simulink model "sbw_data_flow_12_1"  (Simulink 5.0)
settings: Solver=ode45  StartTime=0.0  StopTime=10.0  RelTol=1e-3
settings Model: LastModifiedBy=sandeep

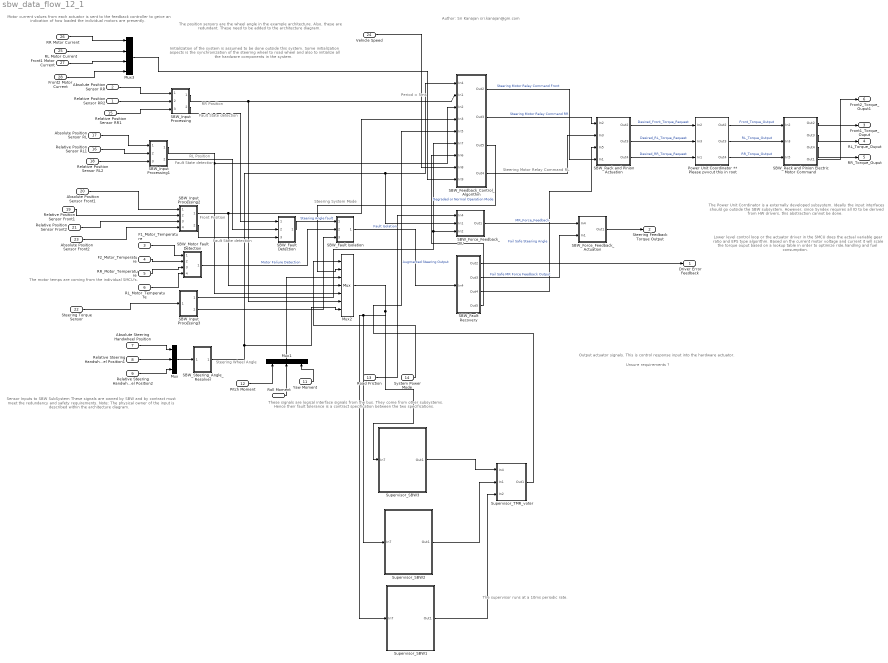
== system sbw_data_flow_12_1 ==
  note: The position sensors are the wheel angle in the example
      | architecture. Also, these are redundant. These need to be added to the architecture
      | diagram.
  note: Sensor Inputs to SBW SubSystem
      | These signals are owned by SBW and by
      | contract must meet the redundancy and safety requirements.
      | Note: The physical
      | owner of the input is described within
      | the architecture diagram.
  note: The motor temps
      | are coming from the
      | individual SMCU's.
  note: These signals are logical interface signals from the bus.
      | They come from other subsystems. Hence their fault tolerance
      | is a contract specification between the two specifications.
  note: Output actuator signals. This is control response
      | input into the hardware actuator.
  note: Steering Wheel Angle
  note: RR Position
  note: RL Position
  note: Front Position
  note: Fault State detection
  note: Fault State detection
  note: Fault State detection
  note: Steering System Mode
  note: Period = 5ms
  note: Steering Motor Relay Command RL
  note: Initialization of the system is assumed to be done outside this system.
      | Some initialization aspects is the synchronization of the steering wheel to
      | road wheel and also to initialize all the hardware components in the system.
  note: The Power Unit Corrdinator is a externally developed
      | subsystem. Ideally the input interfaces should go outside the SBW subsystem.
      | However, since Syndex requires all IO to be derived from HW drivers, this abstraction
      | cannot be done.
  note: Unsure requirements ?
  note: Lower level control loop or the actuator driver in the SMCU
      | does the actual variable gear ratio and EPS type algorithm. Based
      | on the current motor voltage and current it will scale the torque ouput based
      | on a lookup table in order to optimize ride,handling and fuel consumption.
  note: The supervisor runs at
      | a 10ms periodic rate.
  note: Motor current values from each
      | actuator is sent to the feedback controller
      | to geive an indication of how loaded the individual
      | motors are presently.
  note: Author: Sri Kanajan
      | sri.kanajan@gm.com
  Relative Position Sensor RR2 : Inport
  Absolute Position Sensor RR : Inport  Port=2
  F1_Motor_Temperature : Inport  Port=3
  F2_Motor_Temperature : Inport  Port=4
  RR_Motor_Temperature : Inport  Port=5
  RL_Motor_Temperature : Inport  Port=6
  Absolute Steering Handwheel Position : Inport  Port=7
  Relative Steering Handwheel Position1 : Inport  Port=8
  Relative Steering Handwheel Position2 : Inport  Port=9
  Roll Moment : Inport  Port=10
  Yaw Moment : Inport  Port=11
  Pitch Moment : Inport  Port=12
  Road Friction : Inport  Port=13
  System Power Mode : Inport  Port=14
  Relative Position Sensor RR1 : Inport  Port=15
  Relative Position Sensor RL1 : Inport  Port=16
  Absolute Position Sensor RL : Inport  Port=17
  Relative Position Sensor RL2 : Inport  Port=18
  Relative Position Sensor Front1 : Inport  Port=19
  Absolute Position Sensor Front1 : Inport  Port=20
  Relative Position Sensor Front2 : Inport  Port=21
  Steering Torque Sensor : Inport  Port=22
  Absolute Position Sensor Front2 : Inport  Port=23
  Vehicle Speed : Inport  Port=24
  RL Motor Current : Inport  Port=25
  RR Motor Current : Inport  Port=26
  Front1 Motor Current : Inport  Port=27
  Front2 Motor Current : Inport  Port=28
  Mux : Mux  Inputs=3
  Mux1 : Mux  Orientation=up  Inputs=3
  Mux2 : Mux  Inputs=7
  Mux3 : Mux
  Power Unit Coordinator ** Please pvvcut this in root : Subsystem
  SBW_Fault Detection : Subsystem
  SBW_Fault Isolation : Subsystem
  SBW_Fault Recovery : Subsystem
  SBW_Feedback_Control_Algorithm : Subsystem
  SBW_Force_Feedback_Actuation : Subsystem
  SBW_Force_Feedback_DIU : Subsystem
  SBW_Input Processing : Subsystem
  SBW_Input Processing1 : Subsystem
  SBW_Input Processing2 : Subsystem
  SBW_Input Processing3 : Subsystem
  SBW_Motor Fault Detection : Subsystem
  SBW_Rack and Pinion Actuation : Subsystem
  SBW_Rack and Pinion Electric Motor Command : Subsystem
  SBW_Steering_Angle_Resolver : Subsystem
  Supervisor_SBW1 : Subsystem
  Supervisor_SBW2 : Subsystem
  Supervisor_SBW3 : Subsystem
  Supervisor_TMR_voter : Subsystem
  Driver Error Feedback : Outport
  Steering Feedback Torque Output : Outport  Port=2
  Front1_Torque_Ouput : Outport  Port=3
  RL_Torque_Ouput : Outport  Port=4
  RR_Torque_Ouput : Outport  Port=5
  Front2_Torque_Ouput1 : Outport  Port=6
  wires:
  Absolute Steering Handwheel Position/1 -> Mux/1
  Relative Steering Handwheel Position1/1 -> Mux/2
  Relative Steering Handwheel Position2/1 -> Mux/3
  Absolute Position Sensor RR/1 -> SBW_Input Processing/1(In4)
  Relative Position Sensor RR2/1 -> SBW_Input Processing/2(In5)
  F1_Motor_Temperature/1 -> SBW_Motor Fault Detection/1(In4)
  F2_Motor_Temperature/1 -> SBW_Motor Fault Detection/2(In5)
  RR_Motor_Temperature/1 -> SBW_Motor Fault Detection/3(In1)
  RL_Motor_Temperature/1 -> SBW_Motor Fault Detection/4(In2)
  Mux/1 -> SBW_Steering_Angle_Resolver/1(In4)
  Relative Position Sensor RR1/1 -> SBW_Input Processing/3(In1)
  Absolute Position Sensor RL/1 -> SBW_Input Processing1/1(In4)
  Relative Position Sensor RL1/1 -> SBW_Input Processing1/2(In5)
  Relative Position Sensor RL2/1 -> SBW_Input Processing1/3(In1)
  Absolute Position Sensor Front1/1 -> SBW_Input Processing2/1(In4)
  Relative Position Sensor Front1/1 -> SBW_Input Processing2/2(In5)
  Relative Position Sensor Front2/1 -> SBW_Input Processing2/3(In1)
  SBW_Steering_Angle_Resolver/1(Out1) -> SBW_Feedback_Control_Algorithm/1(In4), SBW_Force_Feedback_DIU/2(In1), Mux2/7
  SBW_Input Processing/1(Out1) -> SBW_Feedback_Control_Algorithm/2(In1), Mux2/6
  SBW_Input Processing1/1(Out1) -> Mux2/5, SBW_Feedback_Control_Algorithm/3(In2)
  SBW_Input Processing2/1(Out1) -> SBW_Feedback_Control_Algorithm/4(In3), Mux2/4
  SBW_Force_Feedback_DIU/1(Out1) -> SBW_Force_Feedback_Actuation/1(In4)  "MR_Force_Feedback"
  SBW_Input Processing2/2(Out2) -> SBW_Fault Detection/3(In1)
  SBW_Input Processing/2(Out2) -> SBW_Fault Detection/1(In4)
  SBW_Input Processing1/2(Out2) -> SBW_Fault Detection/2(In5)
  Road Friction/1 -> SBW_Force_Feedback_DIU/1(In4)
  System Power Mode/1 -> Mux2/1
  SBW_Feedback_Control_Algorithm/2(Out3) -> SBW_Rack and Pinion Actuation/1(In2)  "Steering Motor Relay Command RR"
  SBW_Fault Detection/1(Out1) -> SBW_Fault Isolation/1(In4)  "Steering Angle fault"
  SBW_Motor Fault Detection/1(Out1) -> SBW_Fault Isolation/2(In5)  "Motor Faliure Detection"
  SBW_Fault Isolation/1(Out1) -> SBW_Fault Recovery/1(In4)  "Fault Isolation"
  SBW_Fault Recovery/1(Out2) -> Driver Error Feedback/1
  SBW_Feedback_Control_Algorithm/3(Out5) -> Mux2/2
  SBW_Fault Recovery/2(Out3) -> SBW_Force_Feedback_Actuation/2(In1)  "Fail Safe MR Force Feedback Output"
  SBW_Fault Recovery/3(Out4) -> SBW_Rack and Pinion Actuation/3(In5)  "Fail Safe Steering Angle"
  SBW_Force_Feedback_Actuation/1(Out1) -> Steering Feedback Torque Output/1
  SBW_Feedback_Control_Algorithm/4(Out4) -> SBW_Rack and Pinion Actuation/2(In3)
  SBW_Feedback_Control_Algorithm/1(Out2) -> SBW_Rack and Pinion Actuation/4(In1)  "Steering Motor Relay Command Front"
  SBW_Rack and Pinion Actuation/3(Out4) -> Power Unit Coordinator ** Please pvvcut this in root/3(In1)  "Desired_RR_Torque_Request"
  SBW_Rack and Pinion Actuation/2(Out3) -> Power Unit Coordinator ** Please pvvcut this in root/2(In3)  "Desired_RL_Torque_Request"
  SBW_Rack and Pinion Actuation/1(Out2) -> Power Unit Coordinator ** Please pvvcut this in root/1(In2)  "Desired_Front_Torque_Request"
  Power Unit Coordinator ** Please pvvcut this in root/2(Out3) -> SBW_Rack and Pinion Electric Motor Command/2(In3)  "RL_Torque_Output"
  Power Unit Coordinator ** Please pvvcut this in root/3(Out4) -> SBW_Rack and Pinion Electric Motor Command/3(In5)  "RR_Torque_Output"
  SBW_Rack and Pinion Electric Motor Command/1(Out2) -> Front1_Torque_Ouput/1
  Power Unit Coordinator ** Please pvvcut this in root/1(Out2) -> SBW_Rack and Pinion Electric Motor Command/1(In2)  "Front_Torque_Output"
  SBW_Rack and Pinion Electric Motor Command/2(Out3) -> RL_Torque_Ouput/1
  SBW_Rack and Pinion Electric Motor Command/3(Out4) -> RR_Torque_Ouput/1
  Absolute Position Sensor Front2/1 -> SBW_Input Processing2/4(In2)
  Pitch Moment/1 -> Mux1/1
  Roll Moment/1 -> Mux1/2
  Yaw Moment/1 -> Mux1/3
  Mux1/1 -> Mux2/3
  SBW_Rack and Pinion Electric Motor Command/4(Out1) -> Front2_Torque_Ouput1/1
  Mux2/1 -> Supervisor_SBW3/1(In7), Supervisor_SBW2/1(In7), Supervisor_SBW1/1(In7)
  Supervisor_SBW3/1(Out1) -> Supervisor_TMR_voter/1(In4)
  Supervisor_SBW2/1(Out1) -> Supervisor_TMR_voter/2(In1)
  Supervisor_SBW1/1(Out1) -> Supervisor_TMR_voter/3(In2)
  Supervisor_TMR_voter/1(Out1) -> SBW_Feedback_Control_Algorithm/5(In5)  "Augmented Steering Output"
  SBW_Fault Recovery/4(Out5) -> SBW_Feedback_Control_Algorithm/7(In6)  "Degraded or Normal Operation Mode"
  SBW_Input Processing3/1(Out1) -> SBW_Feedback_Control_Algorithm/6(In7), SBW_Force_Feedback_DIU/3(In2)
  SBW_Input Processing3/2(Out2) -> SBW_Fault Isolation/3(In1)
  Steering Torque Sensor/1 -> SBW_Input Processing3/1(In1)
  Vehicle Speed/1 -> SBW_Feedback_Control_Algorithm/8(In8)
  RR Motor Current/1 -> Mux3/1
  RL Motor Current/1 -> Mux3/2
  Front1 Motor Current/1 -> Mux3/3
  Front2 Motor Current/1 -> Mux3/4
  Mux3/1 -> SBW_Feedback_Control_Algorithm/9(In9)

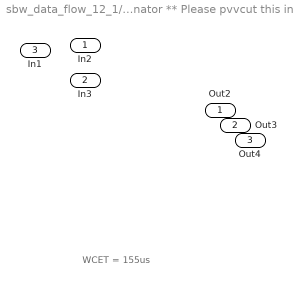
== system sbw_data_flow_12_1/Power Unit Coordinator ** Please pvvcut this in root ==
  note: WCET = 155us
  In2 : Inport
  In3 : Inport  Port=2
  In1 : Inport  Port=3
  Out2 : Outport
  Out3 : Outport  Port=2
  Out4 : Outport  Port=3

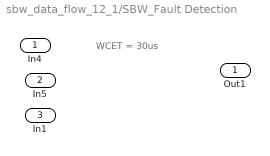
== system sbw_data_flow_12_1/SBW_Fault Detection ==
  note: WCET = 30us
  In4 : Inport
  In5 : Inport  Port=2
  In1 : Inport  Port=3
  Out1 : Outport

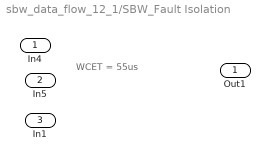
== system sbw_data_flow_12_1/SBW_Fault Isolation ==
  note: WCET = 55us
  In4 : Inport
  In5 : Inport  Port=2
  In1 : Inport  Port=3
  Out1 : Outport

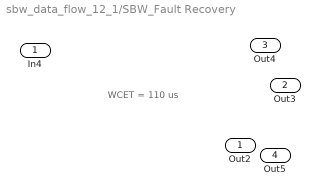
== system sbw_data_flow_12_1/SBW_Fault Recovery ==
  note: WCET = 110 us
  In4 : Inport
  Out2 : Outport
  Out3 : Outport  Port=2
  Out4 : Outport  Port=3
  Out5 : Outport  Port=4

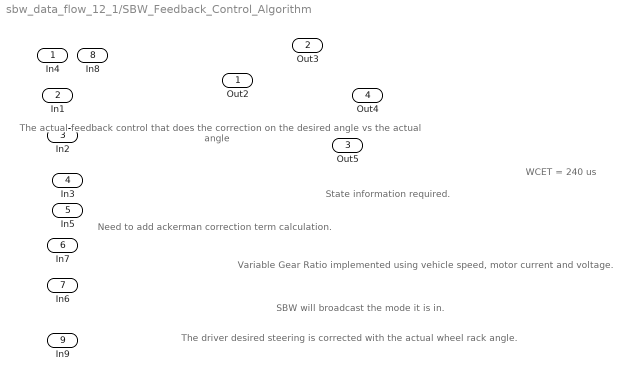
== system sbw_data_flow_12_1/SBW_Feedback_Control_Algorithm ==
  note: The actual feedback control
      | that does the correction on the
      | desired angle vs the actual angle
  note: Need to add ackerman correction
      | term calculation.
  note: State information required.
  note: WCET = 240 us
  note: SBW will broadcast the mode it is in.
  note: The driver desired steering is corrected
      | with the actual wheel rack angle.
  note: Variable Gear Ratio implemented using vehicle speed, motor current and voltage.
  In4 : Inport
  In1 : Inport  Port=2
  In2 : Inport  Port=3
  In3 : Inport  Port=4
  In5 : Inport  Port=5
  In7 : Inport  Port=6
  In6 : Inport  Port=7
  In8 : Inport  Port=8
  In9 : Inport  Port=9
  Out2 : Outport
  Out3 : Outport  Port=2
  Out5 : Outport  Port=3
  Out4 : Outport  Port=4

== system sbw_data_flow_12_1/SBW_Force_Feedback_Actuation ==
  note: WCET = 55us
  In4 : Inport
  In1 : Inport  Port=2
  Out1 : Outport

== system sbw_data_flow_12_1/SBW_Force_Feedback_DIU ==
  note: WCET = 190us
  In4 : Inport
  In1 : Inport  Port=2
  In2 : Inport  Port=3
  Out1 : Outport

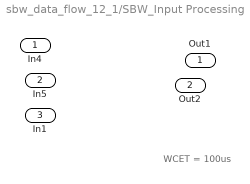
== system sbw_data_flow_12_1/SBW_Input Processing ==
  note: WCET = 100us
  In4 : Inport
  In5 : Inport  Port=2
  In1 : Inport  Port=3
  Out1 : Outport
  Out2 : Outport  Port=2

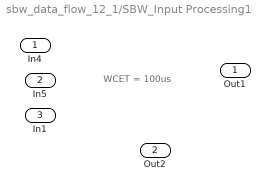
== system sbw_data_flow_12_1/SBW_Input Processing1 ==
  note: WCET = 100us
  In4 : Inport
  In5 : Inport  Port=2
  In1 : Inport  Port=3
  Out1 : Outport
  Out2 : Outport  Port=2

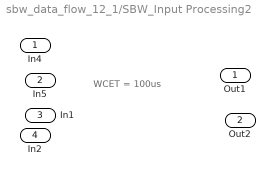
== system sbw_data_flow_12_1/SBW_Input Processing2 ==
  note: WCET = 100us
  In4 : Inport
  In5 : Inport  Port=2
  In1 : Inport  Port=3
  In2 : Inport  Port=4
  Out1 : Outport
  Out2 : Outport  Port=2

== system sbw_data_flow_12_1/SBW_Input Processing3 ==
  note: WCET = 100us
  In1 : Inport
  Out1 : Outport
  Out2 : Outport  Port=2

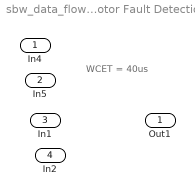
== system sbw_data_flow_12_1/SBW_Motor Fault Detection ==
  note: WCET = 40us
  In4 : Inport
  In5 : Inport  Port=2
  In1 : Inport  Port=3
  In2 : Inport  Port=4
  Out1 : Outport

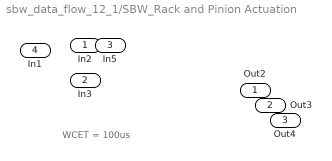
== system sbw_data_flow_12_1/SBW_Rack and Pinion Actuation ==
  note: WCET = 100us
  In2 : Inport
  In3 : Inport  Port=2
  In5 : Inport  Port=3
  In1 : Inport  Port=4
  Out2 : Outport
  Out3 : Outport  Port=2
  Out4 : Outport  Port=3

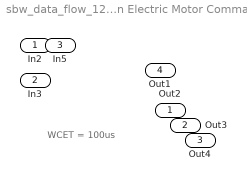
== system sbw_data_flow_12_1/SBW_Rack and Pinion Electric Motor Command ==
  note: WCET = 100us
  In2 : Inport
  In3 : Inport  Port=2
  In5 : Inport  Port=3
  Out2 : Outport
  Out3 : Outport  Port=2
  Out4 : Outport  Port=3
  Out1 : Outport  Port=4

== system sbw_data_flow_12_1/SBW_Steering_Angle_Resolver ==
  note: WCET = 100us
  In4 : Inport
  Out1 : Outport

== system sbw_data_flow_12_1/Supervisor_SBW1 ==
  note: Need to add brake with steering
      | and moding with respect to faults.
  note: WCET = 250 us
  note: Req:
      | The steering mode will inform the supervisor if any
      | augmentation is required.
  note: Has 2 shutdown roles.
  In7 : Inport
  Out1 : Outport

== system sbw_data_flow_12_1/Supervisor_SBW2 ==
  note: Has 2 shutdown roles.
  note: Req:
      | The steering mode will inform the supervisor if any
      | augmentation is required.
  note: WCET = 50 us
  note: Need to add brake with steering
      | and moding with respect to faults.
  In7 : Inport
  Out1 : Outport

== system sbw_data_flow_12_1/Supervisor_SBW3 ==
  note: Has 2 shutdown roles.
      | 1. All supervisor replica's vote to shutdown the rack actuator if
      | it sees that the SMCU is no longer functioning properly.
      | 2. It votes to engage the mechanical backup in the case that the
      | sensor modules disagree or fail.
  note: Req:
      | The steering mode will inform the supervisor if any
      | augmentation is required.
  note: WCET = 250 us
  note: Need to add brake with steering
      | and moding with respect to faults.
  In7 : Inport
  Out1 : Outport

== system sbw_data_flow_12_1/Supervisor_TMR_voter ==
  note: WCET = 30us
  In4 : Inport
  In1 : Inport  Port=2
  In2 : Inport  Port=3
  Out1 : Outport
